simulink model "SS_MMC_dynamic_phasor_small_signal"  (R2023b)
settings: Solver=VariableStepAuto  StartTime=0.0  StopTime=10.0  RelTol=1e-3
settings Model: Creator=dli313  LastModifiedBy=dongyuli

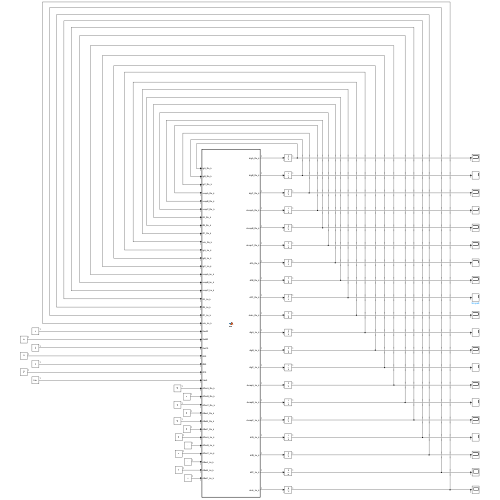
[thumbnail: Simulink's stored preview of the top-level diagram]
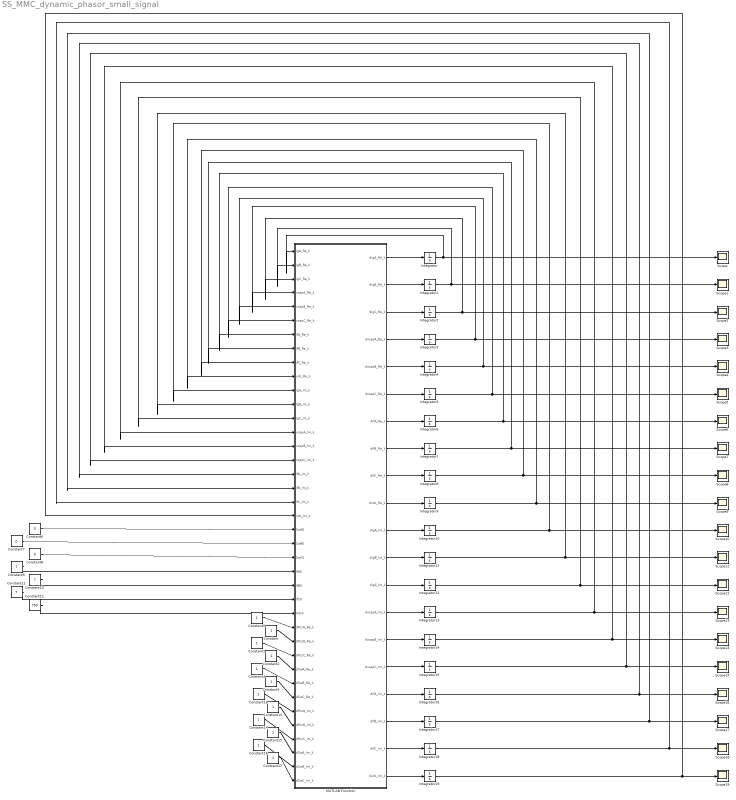
== system SS_MMC_dynamic_phasor_small_signal ==
  Constant{,1..5,13..18} (12 alike) : Constant
  Constant10 : Constant  Value=7
  Constant11 : Constant  Value=7
  Constant12 : Constant  Value=750
  Constant6 : Constant  Value=0
  Constant7 : Constant  Value=0
  Constant8 : Constant  Value=0
  Constant9 : Constant  Value=7
  Integrator{,1..19} (20 alike) : Integrator
  MATLAB Function : MATLAB Function  TreatAsAtomicUnit=on
  Scope{,1..19} (20 alike) : Scope
  wires:
  Constant6/1 -> MATLAB Function/21(SwA0)
  Constant7/1 -> MATLAB Function/22(SwB0)
  Constant8/1 -> MATLAB Function/23(SwC0)
  Constant9/1 -> MATLAB Function/24(ifA0)
  Constant10/1 -> MATLAB Function/25(ifB0)
  Constant11/1 -> MATLAB Function/26(ifC0)
  Constant12/1 -> MATLAB Function/27(Vdc0)
  MATLAB Function/1(digA_Re_k) -> Integrator/1
  MATLAB Function/2(digB_Re_k) -> Integrator1/1
  MATLAB Function/3(digC_Re_k) -> Integrator2/1
  MATLAB Function/4(dvcapA_Re_k) -> Integrator3/1
  MATLAB Function/5(dvcapB_Re_k) -> Integrator4/1
  MATLAB Function/6(dvcapC_Re_k) -> Integrator5/1
  MATLAB Function/7(difA_Re_k) -> Integrator6/1
  MATLAB Function/8(difB_Re_k) -> Integrator7/1
  MATLAB Function/9(difC_Re_k) -> Integrator8/1
  MATLAB Function/10(dvdc_Re_k) -> Integrator9/1
  MATLAB Function/11(digA_Im_k) -> Integrator10/1
  MATLAB Function/12(digB_Im_k) -> Integrator11/1
  MATLAB Function/13(digC_Im_k) -> Integrator12/1
  MATLAB Function/14(dvcapA_Im_k) -> Integrator13/1
  MATLAB Function/20(dvdc_Im_k) -> Integrator19/1
  MATLAB Function/19(difC_Im_k) -> Integrator18/1
  MATLAB Function/18(difB_Im_k) -> Integrator17/1
  MATLAB Function/17(difA_Im_k) -> Integrator16/1
  MATLAB Function/16(dvcapC_Im_k) -> Integrator15/1
  MATLAB Function/15(dvcapB_Im_k) -> Integrator14/1
  Integrator/1 -> Scope/1, MATLAB Function/1(igA_Re_k)
  Integrator1/1 -> Scope1/1, MATLAB Function/2(igB_Re_k)
  Integrator2/1 -> Scope2/1, MATLAB Function/3(igC_Re_k)
  Integrator3/1 -> Scope3/1, MATLAB Function/4(vcapA_Re_k)
  Integrator4/1 -> Scope4/1, MATLAB Function/5(vcapB_Re_k)
  Integrator5/1 -> Scope5/1, MATLAB Function/6(vcapC_Re_k)
  Integrator6/1 -> Scope6/1, MATLAB Function/7(ifA_Re_k)
  Integrator7/1 -> MATLAB Function/8(ifB_Re_k), Scope7/1
  Integrator8/1 -> Scope8/1, MATLAB Function/9(ifC_Re_k)
  Integrator9/1 -> Scope9/1, MATLAB Function/10(vdc_Re_k)
  Integrator10/1 -> Scope10/1, MATLAB Function/11(igA_Im_k)
  Integrator11/1 -> Scope11/1, MATLAB Function/12(igB_Im_k)
  Integrator12/1 -> Scope12/1, MATLAB Function/13(igC_Im_k)
  Integrator15/1 -> Scope15/1, MATLAB Function/16(vcapC_Im_k)
  Integrator16/1 -> Scope16/1, MATLAB Function/17(ifA_Im_k)
  Integrator17/1 -> Scope17/1, MATLAB Function/18(ifB_Im_k)
  Integrator18/1 -> Scope18/1, MATLAB Function/19(ifC_Im_k)
  Integrator19/1 -> Scope19/1, MATLAB Function/20(vdc_Im_k)
  Integrator13/1 -> MATLAB Function/14(vcapA_Im_k), Scope13/1
  Integrator14/1 -> MATLAB Function/15(vcapB_Im_k), Scope14/1
  Constant5/1 -> MATLAB Function/28(dPccA_Re_k)
  Constant/1 -> MATLAB Function/29(dPccB_Re_k)
  Constant1/1 -> MATLAB Function/30(dPccC_Re_k)
  Constant2/1 -> MATLAB Function/31(dSwA_Re_k)
  Constant3/1 -> MATLAB Function/32(dSwB_Re_k)
  Constant4/1 -> MATLAB Function/33(dSwC_Re_k)
  Constant17/1 -> MATLAB Function/39(dSwC_Im_k)
  Constant16/1 -> MATLAB Function/38(dSwB_Im_k)
  Constant14/1 -> MATLAB Function/36(dPccC_Im_k)
  Constant18/1 -> MATLAB Function/34(dPccA_Im_k)
  Constant15/1 -> MATLAB Function/37(dSwA_Im_k)
  Constant13/1 -> MATLAB Function/35(dPccB_Im_k)

== matlab function SS_MMC_dynamic_phasor_small_signal/MATLAB Function ==
  data: igA_Re_k input; digA_Re_k output; digB_Re_k output; digC_Re_k output; dvcapA_Re_k output; dvcapB_Re_k output; dvcapC_Re_k output; difA_Re_k output; difB_Re_k output; difC_Re_k output; dvdc_Re_k output; digA_Im_k output; digB_Im_k output; igB_Re_k input; igC_Re_k input; vcapA_Re_k input; vcapB_Re_k input; vcapC_Re_k input; ifA_Re_k input; ifB_Re_k input; ifC_Re_k input; vdc_Re_k input; igA_Im_k input; igB_Im_k input; igC_Im_k input; vcapA_Im_k input; vcapB_Im_k input; vcapC_Im_k input; ifA_Im_k input; ifB_Im_k input; ifC_Im_k input; vdc_Im_k input; SwA0 input; SwB0 input; SwC0 input; ifA0 input; ifB0 input; ifC0 input; Vdc0 input; digC_Im_k output; dvcapA_Im_k output; dvcapB_Im_k output; dvcapC_Im_k output; difA_Im_k output; difB_Im_k output; difC_Im_k output; dvdc_Im_k output; dPccA_Re_k input; dPccB_Re_k input; dPccC_Re_k input; dSwA_Re_k input; dSwB_Re_k input; dSwC_Re_k input; dPccA_Im_k input; dPccB_Im_k input; dPccC_Im_k input; dSwA_Im_k input; dSwB_Im_k input; dSwC_Im_k input
function [digA_Re_k,  digB_Re_k,  digC_Re_k,  dvcapA_Re_k,  dvcapB_Re_k,  dvcapC_Re_k,  difA_Re_k,  difB_Re_k,  difC_Re_k,  dvdc_Re_k,  digA_Im_k,  digB_Im_k,  digC_Im_k,  dvcapA_Im_k,  dvcapB_Im_k,  dvcapC_Im_k,  difA_Im_k,  difB_Im_k,  difC_Im_k,  dvdc_Im_k]  = fcn(igA_Re_k, igB_Re_k, igC_Re_k, vcapA_Re_k, vcapB_Re_k, vcapC_Re_k, ifA_Re_k, ifB_Re_k, ifC_Re_k, vdc_Re_k, igA_Im_k, igB_Im_k, igC_Im_k, vcapA_Im_k, vcapB_Im_k, vcapC_Im_k, ifA_Im_k, ifB_Im_k, ifC_Im_k, vdc_Im_k, SwA0, SwB0, SwC0, ifA0, ifB0, ifC0, Vdc0, dPccA_Re_k, dPccB_Re_k, dPccC_Re_k, dSwA_Re_k, dSwB_Re_k, dSwC_Re_k, dPccA_Im_k, dPccB_Im_k, dPccC_Im_k, dSwA_Im_k, dSwB_Im_k, dSwC_Im_k)

f = 50;

w = 2*pi*f;

RgA = 1;
RgB = 1;
RgC = 1;

RfA = 0.5;
RfB = 0.5;
RfC = 0.5;

RcfA = 0.5;
RcfB = 0.5;
RcfC = 0.5;

LgA = 3.3e-3;
LgB = 3.3e-3;
LgC = 3.3e-3;

LfA = 6.25e-3;
LfB = 6.25e-3;
LfC = 6.25e-3;

CfA = 94e-6;
CfB = 94e-6;
CfC = 94e-6;

Rdc = 0.01;
Cdc = 450e-6;

A = [(-RgA-RcfA)/LgA 0 0 -1/LgA 0 0 RcfA/LgA 0 0 0;
     0 (-RgB-RcfB)/LgB 0 0 -1/LgB 0 0 RcfB/LgB 0 0;
     0 0 (-RgC-RcfC)/LgC 0 0 -1/LgC 0 0 RcfC/LgC 0;
     1/CfA 0 0 0 0 0 -1/CfA 0 0 0;
     0 1/CfA 0 0 0 0 0 -1/CfB 0 0;
     0 0 1/CfC 0 0 0 0 0 -1/CfC 0;
     RcfA 0 0 1/LfA 0 0 (-RcfA-RfA)/LfA 0 0 -SwA0/LfA;
     0 RcfB/LfB 0 0 1/LfB 0 0 (-RfB-RfB)/LfB 0 -SwB0/LfB;
     0 0 RcfC/LfC 0 0 1/LfC 0 0 (-RcfC-RfC)/LfC -SwC0/LfC;
     0 0 0 0 0 0 SwA0/Cdc SwB0/Cdc SwC0/Cdc -1/(Rdc*Cdc)];

B = [1/LgA 0 0 0 0 0;
    0 1/LgB 0 0 0 0;
    0 0 1/LgC 0 0 0;
    0 0 0 0 0 0;
    0 0 0 0 0 0;
    0 0 0 0 0 0;
    0 0 0 -Vdc0/LfA 0 0;
    0 0 0 0 -Vdc0/LfB 0;
    0 0 0 0 0 -Vdc0/LfC;
    0 0 0 ifA0/Cdc ifB0/Cdc ifC0/Cdc];

X = [igA_Re_k, igB_Re_k, igC_Re_k, vcapA_Re_k, vcapB_Re_k, vcapC_Re_k, ifA_Re_k, ifB_Re_k, ifC_Re_k, vdc_Re_k, igA_Im_k, igB_Im_k, igC_Im_k, vcapA_Im_k, vcapB_Im_k, vcapC_Im_k, ifA_Im_k, ifB_Im_k, ifC_Im_k, vdc_Im_k]';

k = 1;

I = eye(10);

O = zeros(10,6);

A_k = [A k*w*I;
      -k*w*I A];

B_k = [B O; O B];

U = [dPccA_Re_k, dPccB_Re_k, dPccC_Re_k, dPccA_Im_k, dPccB_Im_k, dPccC_Im_k, dSwA_Re_k, dSwB_Re_k, dSwC_Re_k, dSwA_Im_k, dSwB_Im_k, dSwC_Im_k]';

dX = A_k*X + B_k*U;

digA_Re_k = dX(1);
digB_Re_k = dX(2);
digC_Re_k = dX(3);
dvcapA_Re_k = dX(4);
dvcapB_Re_k = dX(5);
dvcapC_Re_k = dX(6);
difA_Re_k = dX(7);
difB_Re_k = dX(8);
difC_Re_k = dX(9);
dvdc_Re_k = dX(10);

digA_Im_k = dX(11);
digB_Im_k = dX(12);
digC_Im_k = dX(13);
dvcapA_Im_k = dX(14);
dvcapB_Im_k = dX(15);
dvcapC_Im_k = dX(16);
difA_Im_k = dX(17);
difB_Im_k = dX(18);
difC_Im_k = dX(19);
dvdc_Im_k = dX(20);

end
